simulink model "Thandra_Rushikasim_S2lab5"  (R2022a)
settings: Solver=VariableStepAuto  StartTime=0.0  StopTime=1  RelTol=1e-3
libraries: commanapbnd3 x1
settings Model: Creator=rishika  LastModifiedBy=rishika

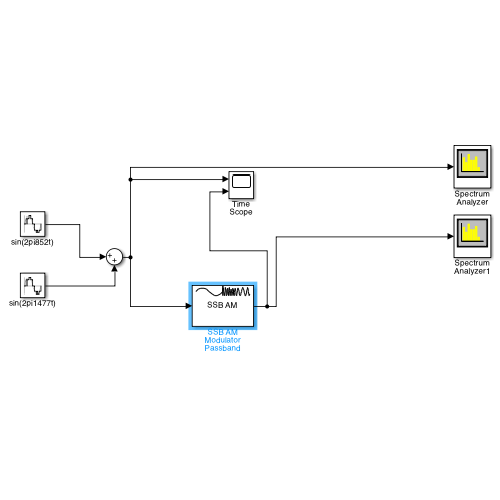
[thumbnail: Simulink's stored preview of the top-level diagram]
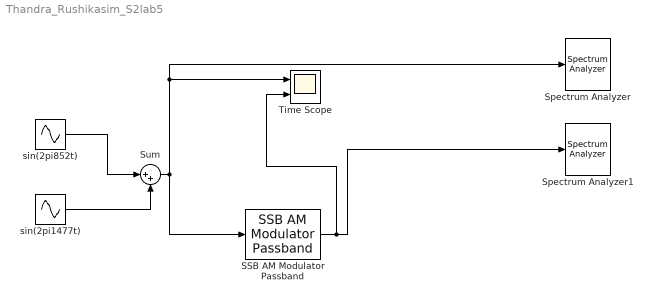
== system Thandra_Rushikasim_S2lab5 ==
  SSB AM Modulator Passband : commanapbnd3/SSB AM Modulator Passband  Fc=8000  Ph=0  Sd=Lower  Ho=100
      settings: SourceProductBaseCode=CM
  Spectrum Analyzer : SpectrumAnalyzer
  Spectrum Analyzer1 : SpectrumAnalyzer
  Sum : Sum  Inputs=|++
  Time Scope : Scope  NumInputPorts=2
  sin(2pi1477t) : Sin  Frequency=2*pi*1477  SampleTime=0.00001
  sin(2pi852t) : Sin  Frequency=2*pi*852  SampleTime=0.00001
  wires:
  sin(2pi1477t)/1 -> Sum/2
  Sum/1 -> SSB AM Modulator Passband/1, Time Scope/1, Spectrum Analyzer/1
  sin(2pi852t)/1 -> Sum/1
  SSB AM Modulator Passband/1 -> Time Scope/2, Spectrum Analyzer1/1
